simulink model "Lab_02_01_3157"  (R2023a)
settings: Solver=VariableStepAuto  StartTime=0.0  StopTime=10.0  RelTol=1e-3
libraries: spsMosfetLib x4, spsCurrentMeasurementLib x3, spsSeriesRLCBranchLib x3, spsVoltageMeasurementLib x2, spsDCVoltageSourceLib x1, spsPVArrayLib x1, spsPWMGeneratorDCDCLib x1, spspowerguiLib x1
settings Model: Creator=leifi  LastModifiedBy=SirM
settings ModelReferenceCC: EnableRefExpFcnMdlSchedulingChecks=on

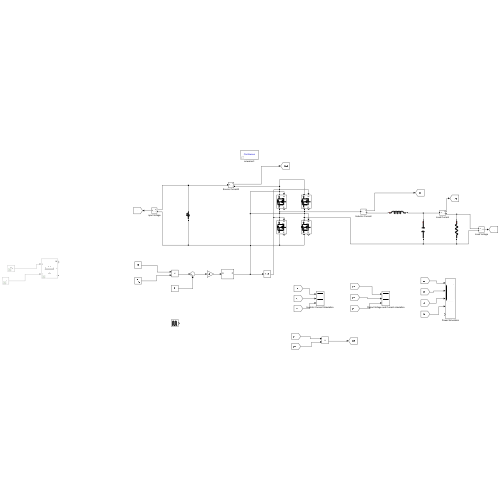
[thumbnail: Simulink's stored preview of the top-level diagram]
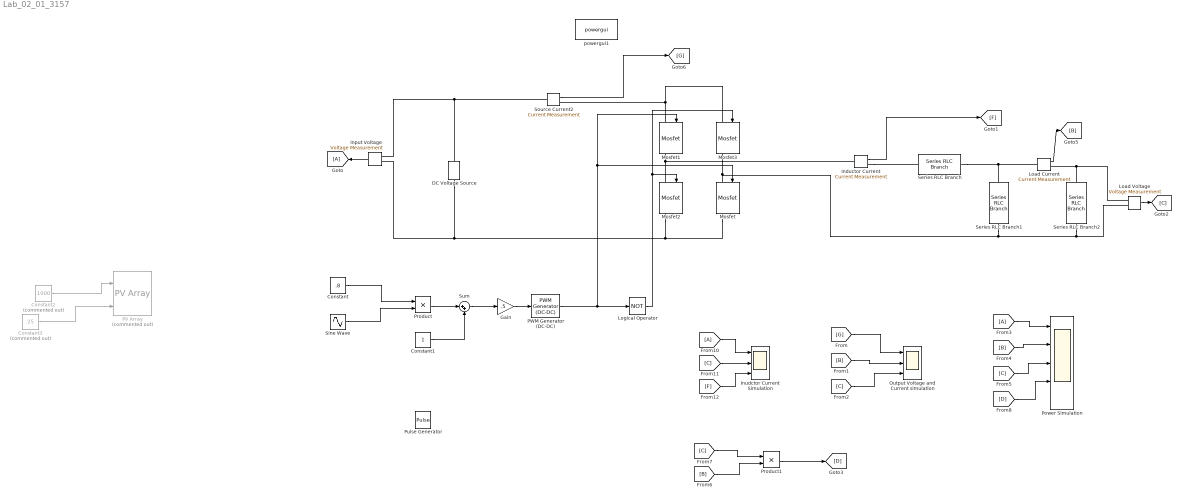
== system Lab_02_01_3157 ==
  Constant : Constant  Value=.8
  Constant1 : Constant
  Constant2 : Constant  Commented=on  Value=1000
  Constant3 : Constant  Commented=on  Value=25
  DC Voltage Source : spsDCVoltageSourceLib/DC Voltage Source  Amplitude=30  Measurements=Voltage
  From10 : From
  From3 : From
  Gain : Gain  Gain=.5
  Goto : Goto
  Inductor Current : spsCurrentMeasurementLib/Current Measurement  PhasorSimulation=off  OutputType=Complex  PSBequivalent=0
  Input Voltage : spsVoltageMeasurementLib/Voltage Measurement  PhasorSimulation=off  OutputType=Complex  PSBequivalent=0
  Inudctor Current Simulation : Scope  NumInputPorts=3
  Load Current : spsCurrentMeasurementLib/Current Measurement  PhasorSimulation=off  OutputType=Complex  PSBequivalent=0
  Load Voltage : spsVoltageMeasurementLib/Voltage Measurement  PhasorSimulation=off  OutputType=Complex  PSBequivalent=0
  Logical Operator : Logic  Operator=NOT  AllPortsSameDT=off  OutDataTypeStr=boolean
  Mosfet{,1..3} (4 alike) : spsMosfetLib/Mosfet  Ron=0.1  Lon=0  Rd=0.01  Vfd=0  IC=0  Rs=1e5  Cs=inf  Measurements=on
  Output Voltage and Current simulation : Scope  NumInputPorts=3
  PV Array : spsPVArrayLib/PV Array  Commented=on  Npar=1  Nser=1  PlotType=array @ 1000 W/m2 & specified temperatures  S_vec="[ 1000  500  100 ]"  Temp_C_vec="[ 45 25  ]"  ModuleName=Amerisolar-Worldwide Energy and Manufacturing USA Co._ Ltd AS-6M-290W  PlotWhenSelected=off  Pm=290.338  Ncell=72  Voc=44.5  Isc=8.68  Vm=35.8  Im=8.11  beta_Voc_pc=-0.39  alpha_Isc_pc=0.04  beta_Voc=-0.17355  alpha_Isc=0.003472  IL=8.7103  I0=7.7395e-10  nI=1.0402  Rsh=283.6831  Rs=0.38472  RobustModel=off  RobustCellTemperature=313.3991  BAL=on  Tc=1e-6  Tfilter=5e-5
  PWM Generator (DC-DC) : spsPWMGeneratorDCDCLib/PWM Generator (DC-DC)  Fsw=5000  Ts=0
  Power Simulation : Scope  NumInputPorts=5
  Product : Product
  Product1 : Product
  Pulse Generator : DiscretePulseGenerator  PulseType=Time based  Amplitude=100  Period=1/40000  PulseWidth=80
  Series RLC Branch : spsSeriesRLCBranchLib/Series RLC Branch  LConnTagsString=__new0  RConnTagsString=__new0  BranchType=L  Resistance=1  Inductance=25e-6  SetiL0=off  InitialCurrent=0  Capacitance=1e-6  Setx0=off  InitialVoltage=0  Measurements=None
  Series RLC Branch1 : spsSeriesRLCBranchLib/Series RLC Branch  LConnTagsString=__new0  RConnTagsString=__new0  BranchType=C  Resistance=1  Inductance=1e-3  SetiL0=off  InitialCurrent=0  Capacitance=1.25e-6  Setx0=off  InitialVoltage=0  Measurements=None
  Series RLC Branch2 : spsSeriesRLCBranchLib/Series RLC Branch  LConnTagsString=__new0  RConnTagsString=__new0  BranchType=R  Resistance=3  Inductance=1e-3  SetiL0=off  InitialCurrent=0  Capacitance=1e-6  Setx0=off  InitialVoltage=0  Measurements=None
  Sine Wave : Sin  Amplitude=30  Frequency=1/40000  SampleTime=0
  Source Current2 : spsCurrentMeasurementLib/Current Measurement  PhasorSimulation=off  OutputType=Complex  PSBequivalent=0
  Sum : Sum  Inputs=|++
  powergui1 : spspowerguiLib/powergui  Priority=1  SimulationMode=Continuous  SampleTime=50e-6  frequency=60  Iterations=50  frequencyindice=0  Pbase=100e6  ErrMax=1e-4  UnitsV=kV  UnitsW=MW  buscounter=0  FunctionMessages=off  echomessages=off  EnableUseOfTLC=off  CurrentSourceSwitches=off  DisableSnubberDevices=off  DisableRonSwitches=off  DisableVfSwitches=off  DisplayEquations=off  AutomaticDiscreteSolvers=off  SolverType=Tustin/Backward Euler (TBE)  Interpol=off  ExternalGateDelay=off  methode=off  Ts=100  x0status=blocks  SPID=on  SwTol=0  HookPort=off  NonlinearTolerance=1e-4  nMaxIteration=100  ContinueOnMaxIteration=off  RestoreLinks=warning  ResistiveCurrentMeasurement=off  Frange=[0:2:500]  Ylog=off  Xlog=on  ShowGrid=off  save=off  variable=ZData  structure=0  ZoomFFT=off  StartTime=0.0  cycles=1  DisplayStyle=1  fundamental=60  FreqAxis=off  MaxFrequency=1000  frequencyindicesteady=1  RmsSteady=1  display=off
  wires:
  [F] -> Inudctor Current Simulation/3
  [C] -> Inudctor Current Simulation/2
  [D] -> Power Simulation/4
  Inductor Current/1 -> [F]
  [B] -> Power Simulation/2
  Load Current/1 -> [B]
  [B] -> Output Voltage and Current simulation/2
  From3/1 -> Power Simulation/1
  Load Voltage/1 -> [C]
  [C] -> Power Simulation/3
  [C] -> Output Voltage and Current simulation/3
  [G] -> Output Voltage and Current simulation/1
  Input Voltage/1 -> Goto/1
  From10/1 -> Inudctor Current Simulation/1
  Logical Operator/1 -> Mosfet3/1, Mosfet2/1
  PWM Generator (DC-DC)/1 -> Logical Operator/1, Mosfet1/1, Mosfet/1
  Gain/1 -> PWM Generator (DC-DC)/1
  Constant1/1 -> Sum/2
  Constant/1 -> Product/1
  Sine Wave/1 -> Product/2
  Source Current2/1 -> [G]
  Constant2/1 -> PV Array/1
  Constant3/1 -> PV Array/2
  Product/1 -> Sum/1
  Sum/1 -> Gain/1
  [C] -> Product1/1
  [B] -> Product1/2
  Product1/1 -> [D]
  connections:
  Series RLC Branch2/LConn1 -- Load Voltage/LConn1 -- Load Current/RConn1
  Series RLC Branch1/RConn1 -- Load Voltage/LConn2 -- Series RLC Branch2/RConn1 -- Mosfet3/RConn1 -- Mosfet/LConn1
  Mosfet1/RConn1 -- Inductor Current/LConn1 -- Mosfet2/LConn1
  Series RLC Branch/RConn1 -- Load Current/LConn1 -- Series RLC Branch1/LConn1
  Mosfet2/RConn1 -- DC Voltage Source/LConn1 -- Input Voltage/LConn2 -- Mosfet/RConn1
  Source Current2/LConn1 -- DC Voltage Source/RConn1 -- Input Voltage/LConn1
  Mosfet1/LConn1 -- Mosfet3/LConn1 -- Source Current2/RConn1
  Inductor Current/RConn1 -- Series RLC Branch/LConn1
